simulink model "c960x4096_x14_7_r2013b_frb"  (R2013b)
settings: Solver=ode45  StartTime=0.0  StopTime=40960  RelTol=1e-3
undefined symbols (not defined in the file): sfp
libraries: xbsIndex_r4 x14620, casper_library_misc x61, dspsigops x32, casper_library_multipliers x24, simulink x18, xps_library x18
(part 38 of 79)

== system c960x4096_x14_7_r2013b_frb/vacc/vacc/xx/bit_sel2 ==
  shift : Inport
  sync : Inport  Port=2
  din64 : Inport  Port=3
  Reinterpret : xbsIndex_r4/Reinterpret  force_arith_type=on  arith_type=Unsigned  force_bin_pt=on  bin_pt=0  block_type=reinterpret
  barrel_switcher : Subsystem  AncestorBlock=casper_library_reorder/barrel_switcher  mask(barrel_switcher){n_inputs=6, async=off}
      mask prompts: n_inputs "Number of Inputs: (2^?)"; async "Asynchronous operation"
      mask help:
      | Shifts input to right by amount specified on sel,
      | wrapping around into higher order bits.
      mask init:
      | barrel_switcher_init(gcb,...
      |     'n_inputs', n_inputs, ...
      |     'async', async);
      mask Help: eval('xlWeb(''http://casper.berkeley.edu/wiki/Barrel_switcher'')')
  bus_create : Subsystem  AncestorBlock=casper_library_flow_control/bus_create  mask(bus_create){inputNum=8}
      mask prompts: inputNum "Number of inputs:"
      mask init:
      | bus_create_init(gcb,...
      |     'inputNum', inputNum);
  bus_expand1 : Subsystem  AncestorBlock=casper_library_flow_control/bus_expand  mask(bus_expand){mode=divisions of equal size, outputNum=64, outputWidth=1, outputBinaryPt=0, outputArithmeticType=0, show_format=off, outputToWorkspace=off, variablePrefix=out, outputToModelAsWell=on}
      mask prompts: outputNum "Number of outputs:"; outputWidth "Output width:"; outputBinaryPt "Output binary point position:"; outputArithmeticType "Output arithmetic type (ufix=0, fix=1, bool=2):"; show_format "Print format string?"; outputToWorkspace "Output to workspace?"; variablePrefix "Variable name prefix:"; outputToModelAsWell "Output to model as well?"
      mask help:
      | Expands a 'bus' made using a bus_create or Xilinx
      | concat block.
      | The input will be divided into the specified number
      | of outputs with the specified arithmetic types.
      | Divisions are made from most significant bit.
      mask init: same as c960x4096_x14_7_r2013b_frb/ssg/bus_expand
      settings: AttributesFormatString=64 outputs
      mask TypeOptions mode: divisions of equal size | divisions of arbitrary size
      mask Callback mode: bus_expand_callback();
      mask Callback outputWidth: bus_expand_callback();
      mask Callback outputToWorkspace: bus_expand_callback();
  sync_out : Outport
  dout16 : Outport  Port=2
  wires:
  bus_expand1/13(out52) -> barrel_switcher/15(In13)
  bus_expand1/42(out23) -> barrel_switcher/44(In42)
  bus_expand1/27(out38) -> barrel_switcher/29(In27)
  bus_expand1/26(out39) -> barrel_switcher/28(In26)
  bus_expand1/33(out32) -> barrel_switcher/35(In33)
  bus_expand1/44(out21) -> barrel_switcher/46(In44)
  bus_expand1/12(out53) -> barrel_switcher/14(In12)
  bus_expand1/35(out30) -> barrel_switcher/37(In35)
  bus_expand1/23(out42) -> barrel_switcher/25(In23)
  bus_expand1/45(out20) -> barrel_switcher/47(In45)
  bus_expand1/50(out15) -> barrel_switcher/52(In50)
  bus_expand1/56(out9) -> barrel_switcher/58(In56)
  sync/1 -> barrel_switcher/2(sync_in)
  bus_expand1/24(out41) -> barrel_switcher/26(In24)
  bus_expand1/58(out7) -> barrel_switcher/60(In58)
  bus_expand1/53(out12) -> barrel_switcher/55(In53)
  bus_expand1/29(out36) -> barrel_switcher/31(In29)
  bus_expand1/43(out22) -> barrel_switcher/45(In43)
  bus_expand1/3(out62) -> barrel_switcher/5(In3)
  bus_expand1/61(out4) -> barrel_switcher/63(In61)
  bus_expand1/1(msb_out64) -> barrel_switcher/3(In1)
  bus_expand1/28(out37) -> barrel_switcher/30(In28)
  Reinterpret/1 -> bus_expand1/1(bus_in)
  bus_expand1/8(out57) -> barrel_switcher/10(In8)
  bus_expand1/20(out45) -> barrel_switcher/22(In20)
  bus_expand1/59(out6) -> barrel_switcher/61(In59)
  bus_expand1/30(out35) -> barrel_switcher/32(In30)
  bus_expand1/19(out46) -> barrel_switcher/21(In19)
  bus_expand1/9(out56) -> barrel_switcher/11(In9)
  bus_expand1/11(out54) -> barrel_switcher/13(In11)
  bus_expand1/18(out47) -> barrel_switcher/20(In18)
  bus_expand1/25(out40) -> barrel_switcher/27(In25)
  bus_expand1/32(out33) -> barrel_switcher/34(In32)
  bus_expand1/62(out3) -> barrel_switcher/64(In62)
  bus_expand1/37(out28) -> barrel_switcher/39(In37)
  bus_expand1/36(out29) -> barrel_switcher/38(In36)
  bus_expand1/41(out24) -> barrel_switcher/43(In41)
  bus_expand1/22(out43) -> barrel_switcher/24(In22)
  bus_expand1/48(out17) -> barrel_switcher/50(In48)
  bus_expand1/7(out58) -> barrel_switcher/9(In7)
  bus_expand1/63(out2) -> barrel_switcher/65(In63)
  bus_expand1/15(out50) -> barrel_switcher/17(In15)
  bus_expand1/49(out16) -> barrel_switcher/51(In49)
  shift/1 -> barrel_switcher/1(sel)
  bus_expand1/21(out44) -> barrel_switcher/23(In21)
  bus_expand1/46(out19) -> barrel_switcher/48(In46)
  bus_expand1/52(out13) -> barrel_switcher/54(In52)
  bus_expand1/54(out11) -> barrel_switcher/56(In54)
  bus_expand1/4(out61) -> barrel_switcher/6(In4)
  bus_expand1/31(out34) -> barrel_switcher/33(In31)
  bus_expand1/40(out25) -> barrel_switcher/42(In40)
  bus_expand1/39(out26) -> barrel_switcher/41(In39)
  bus_expand1/51(out14) -> barrel_switcher/53(In51)
  bus_expand1/64(lsb_out1) -> barrel_switcher/66(In64)
  bus_expand1/38(out27) -> barrel_switcher/40(In38)
  din64/1 -> Reinterpret/1
  bus_expand1/5(out60) -> barrel_switcher/7(In5)
  bus_expand1/17(out48) -> barrel_switcher/19(In17)
  bus_expand1/16(out49) -> barrel_switcher/18(In16)
  bus_expand1/10(out55) -> barrel_switcher/12(In10)
  bus_expand1/14(out51) -> barrel_switcher/16(In14)
  bus_expand1/2(out63) -> barrel_switcher/4(In2)
  bus_expand1/60(out5) -> barrel_switcher/62(In60)
  bus_expand1/55(out10) -> barrel_switcher/57(In55)
  bus_expand1/6(out59) -> barrel_switcher/8(In6)
  bus_expand1/47(out18) -> barrel_switcher/49(In47)
  bus_expand1/57(out8) -> barrel_switcher/59(In57)
  bus_expand1/34(out31) -> barrel_switcher/36(In34)
  barrel_switcher/1(sync_out) -> sync_out/1
  bus_create/1(bus_out) -> dout16/1
  barrel_switcher/58(Out57) -> bus_create/1(in1)
  barrel_switcher/59(Out58) -> bus_create/2(in2)
  barrel_switcher/60(Out59) -> bus_create/3(in3)
  barrel_switcher/61(Out60) -> bus_create/4(in4)
  barrel_switcher/62(Out61) -> bus_create/5(in5)
  barrel_switcher/63(Out62) -> bus_create/6(in6)
  barrel_switcher/64(Out63) -> bus_create/7(in7)
  barrel_switcher/65(Out64) -> bus_create/8(in8)

== system c960x4096_x14_7_r2013b_frb/vacc/vacc/xx/bit_sel3 ==
  shift : Inport
  sync : Inport  Port=2
  din64 : Inport  Port=3
  Reinterpret : xbsIndex_r4/Reinterpret  force_arith_type=on  arith_type=Unsigned  force_bin_pt=on  bin_pt=0  block_type=reinterpret
  barrel_switcher : Subsystem  AncestorBlock=casper_library_reorder/barrel_switcher  mask(barrel_switcher){n_inputs=6, async=off}
      mask prompts: n_inputs "Number of Inputs: (2^?)"; async "Asynchronous operation"
      mask help:
      | Shifts input to right by amount specified on sel,
      | wrapping around into higher order bits.
      mask init:
      | barrel_switcher_init(gcb,...
      |     'n_inputs', n_inputs, ...
      |     'async', async);
      mask Help: eval('xlWeb(''http://casper.berkeley.edu/wiki/Barrel_switcher'')')
  bus_create : Subsystem  AncestorBlock=casper_library_flow_control/bus_create  mask(bus_create){inputNum=8}
      mask prompts: inputNum "Number of inputs:"
      mask init:
      | bus_create_init(gcb,...
      |     'inputNum', inputNum);
  bus_expand1 : Subsystem  AncestorBlock=casper_library_flow_control/bus_expand  mask(bus_expand){mode=divisions of equal size, outputNum=64, outputWidth=1, outputBinaryPt=0, outputArithmeticType=0, show_format=off, outputToWorkspace=off, variablePrefix=out, outputToModelAsWell=on}
      mask prompts: outputNum "Number of outputs:"; outputWidth "Output width:"; outputBinaryPt "Output binary point position:"; outputArithmeticType "Output arithmetic type (ufix=0, fix=1, bool=2):"; show_format "Print format string?"; outputToWorkspace "Output to workspace?"; variablePrefix "Variable name prefix:"; outputToModelAsWell "Output to model as well?"
      mask help:
      | Expands a 'bus' made using a bus_create or Xilinx
      | concat block.
      | The input will be divided into the specified number
      | of outputs with the specified arithmetic types.
      | Divisions are made from most significant bit.
      mask init: same as c960x4096_x14_7_r2013b_frb/ssg/bus_expand
      settings: AttributesFormatString=64 outputs
      mask TypeOptions mode: divisions of equal size | divisions of arbitrary size
      mask Callback mode: bus_expand_callback();
      mask Callback outputWidth: bus_expand_callback();
      mask Callback outputToWorkspace: bus_expand_callback();
  sync_out : Outport
  dout16 : Outport  Port=2
  wires:
  bus_expand1/13(out52) -> barrel_switcher/15(In13)
  bus_expand1/42(out23) -> barrel_switcher/44(In42)
  bus_expand1/27(out38) -> barrel_switcher/29(In27)
  bus_expand1/26(out39) -> barrel_switcher/28(In26)
  bus_expand1/33(out32) -> barrel_switcher/35(In33)
  bus_expand1/44(out21) -> barrel_switcher/46(In44)
  bus_expand1/12(out53) -> barrel_switcher/14(In12)
  bus_expand1/35(out30) -> barrel_switcher/37(In35)
  bus_expand1/23(out42) -> barrel_switcher/25(In23)
  bus_expand1/45(out20) -> barrel_switcher/47(In45)
  bus_expand1/50(out15) -> barrel_switcher/52(In50)
  bus_expand1/56(out9) -> barrel_switcher/58(In56)
  sync/1 -> barrel_switcher/2(sync_in)
  bus_expand1/24(out41) -> barrel_switcher/26(In24)
  bus_expand1/58(out7) -> barrel_switcher/60(In58)
  bus_expand1/53(out12) -> barrel_switcher/55(In53)
  bus_expand1/29(out36) -> barrel_switcher/31(In29)
  bus_expand1/43(out22) -> barrel_switcher/45(In43)
  bus_expand1/3(out62) -> barrel_switcher/5(In3)
  bus_expand1/61(out4) -> barrel_switcher/63(In61)
  bus_expand1/1(msb_out64) -> barrel_switcher/3(In1)
  bus_expand1/28(out37) -> barrel_switcher/30(In28)
  Reinterpret/1 -> bus_expand1/1(bus_in)
  bus_expand1/8(out57) -> barrel_switcher/10(In8)
  bus_expand1/20(out45) -> barrel_switcher/22(In20)
  bus_expand1/59(out6) -> barrel_switcher/61(In59)
  bus_expand1/30(out35) -> barrel_switcher/32(In30)
  bus_expand1/19(out46) -> barrel_switcher/21(In19)
  bus_expand1/9(out56) -> barrel_switcher/11(In9)
  bus_expand1/11(out54) -> barrel_switcher/13(In11)
  bus_expand1/18(out47) -> barrel_switcher/20(In18)
  bus_expand1/25(out40) -> barrel_switcher/27(In25)
  bus_expand1/32(out33) -> barrel_switcher/34(In32)
  bus_expand1/62(out3) -> barrel_switcher/64(In62)
  bus_expand1/37(out28) -> barrel_switcher/39(In37)
  bus_expand1/36(out29) -> barrel_switcher/38(In36)
  bus_expand1/41(out24) -> barrel_switcher/43(In41)
  bus_expand1/22(out43) -> barrel_switcher/24(In22)
  bus_expand1/48(out17) -> barrel_switcher/50(In48)
  bus_expand1/7(out58) -> barrel_switcher/9(In7)
  bus_expand1/63(out2) -> barrel_switcher/65(In63)
  bus_expand1/15(out50) -> barrel_switcher/17(In15)
  bus_expand1/49(out16) -> barrel_switcher/51(In49)
  shift/1 -> barrel_switcher/1(sel)
  bus_expand1/21(out44) -> barrel_switcher/23(In21)
  bus_expand1/46(out19) -> barrel_switcher/48(In46)
  bus_expand1/52(out13) -> barrel_switcher/54(In52)
  bus_expand1/54(out11) -> barrel_switcher/56(In54)
  bus_expand1/4(out61) -> barrel_switcher/6(In4)
  bus_expand1/31(out34) -> barrel_switcher/33(In31)
  bus_expand1/40(out25) -> barrel_switcher/42(In40)
  bus_expand1/39(out26) -> barrel_switcher/41(In39)
  bus_expand1/51(out14) -> barrel_switcher/53(In51)
  bus_expand1/64(lsb_out1) -> barrel_switcher/66(In64)
  bus_expand1/38(out27) -> barrel_switcher/40(In38)
  din64/1 -> Reinterpret/1
  bus_expand1/5(out60) -> barrel_switcher/7(In5)
  bus_expand1/17(out48) -> barrel_switcher/19(In17)
  bus_expand1/16(out49) -> barrel_switcher/18(In16)
  bus_expand1/10(out55) -> barrel_switcher/12(In10)
  bus_expand1/14(out51) -> barrel_switcher/16(In14)
  bus_expand1/2(out63) -> barrel_switcher/4(In2)
  bus_expand1/60(out5) -> barrel_switcher/62(In60)
  bus_expand1/55(out10) -> barrel_switcher/57(In55)
  bus_expand1/6(out59) -> barrel_switcher/8(In6)
  bus_expand1/47(out18) -> barrel_switcher/49(In47)
  bus_expand1/57(out8) -> barrel_switcher/59(In57)
  bus_expand1/34(out31) -> barrel_switcher/36(In34)
  barrel_switcher/1(sync_out) -> sync_out/1
  bus_create/1(bus_out) -> dout16/1
  barrel_switcher/58(Out57) -> bus_create/1(in1)
  barrel_switcher/59(Out58) -> bus_create/2(in2)
  barrel_switcher/60(Out59) -> bus_create/3(in3)
  barrel_switcher/61(Out60) -> bus_create/4(in4)
  barrel_switcher/62(Out61) -> bus_create/5(in5)
  barrel_switcher/63(Out62) -> bus_create/6(in6)
  barrel_switcher/64(Out63) -> bus_create/7(in7)
  barrel_switcher/65(Out64) -> bus_create/8(in8)

== system c960x4096_x14_7_r2013b_frb/vacc/vacc/xx/bit_sel4 ==
  shift : Inport
  sync : Inport  Port=2
  din64 : Inport  Port=3
  Reinterpret : xbsIndex_r4/Reinterpret  force_arith_type=on  arith_type=Unsigned  force_bin_pt=on  bin_pt=0  block_type=reinterpret
  barrel_switcher : Subsystem  AncestorBlock=casper_library_reorder/barrel_switcher  mask(barrel_switcher){n_inputs=6, async=off}
      mask prompts: n_inputs "Number of Inputs: (2^?)"; async "Asynchronous operation"
      mask help:
      | Shifts input to right by amount specified on sel,
      | wrapping around into higher order bits.
      mask init:
      | barrel_switcher_init(gcb,...
      |     'n_inputs', n_inputs, ...
      |     'async', async);
      mask Help: eval('xlWeb(''http://casper.berkeley.edu/wiki/Barrel_switcher'')')
  bus_create : Subsystem  AncestorBlock=casper_library_flow_control/bus_create  mask(bus_create){inputNum=8}
      mask prompts: inputNum "Number of inputs:"
      mask init:
      | bus_create_init(gcb,...
      |     'inputNum', inputNum);
  bus_expand1 : Subsystem  AncestorBlock=casper_library_flow_control/bus_expand  mask(bus_expand){mode=divisions of equal size, outputNum=64, outputWidth=1, outputBinaryPt=0, outputArithmeticType=0, show_format=off, outputToWorkspace=off, variablePrefix=out, outputToModelAsWell=on}
      mask prompts: outputNum "Number of outputs:"; outputWidth "Output width:"; outputBinaryPt "Output binary point position:"; outputArithmeticType "Output arithmetic type (ufix=0, fix=1, bool=2):"; show_format "Print format string?"; outputToWorkspace "Output to workspace?"; variablePrefix "Variable name prefix:"; outputToModelAsWell "Output to model as well?"
      mask help:
      | Expands a 'bus' made using a bus_create or Xilinx
      | concat block.
      | The input will be divided into the specified number
      | of outputs with the specified arithmetic types.
      | Divisions are made from most significant bit.
      mask init: same as c960x4096_x14_7_r2013b_frb/ssg/bus_expand
      settings: AttributesFormatString=64 outputs
      mask TypeOptions mode: divisions of equal size | divisions of arbitrary size
      mask Callback mode: bus_expand_callback();
      mask Callback outputWidth: bus_expand_callback();
      mask Callback outputToWorkspace: bus_expand_callback();
  sync_out : Outport
  dout16 : Outport  Port=2
  wires:
  bus_expand1/13(out52) -> barrel_switcher/15(In13)
  bus_expand1/42(out23) -> barrel_switcher/44(In42)
  bus_expand1/27(out38) -> barrel_switcher/29(In27)
  bus_expand1/26(out39) -> barrel_switcher/28(In26)
  bus_expand1/33(out32) -> barrel_switcher/35(In33)
  bus_expand1/44(out21) -> barrel_switcher/46(In44)
  bus_expand1/12(out53) -> barrel_switcher/14(In12)
  bus_expand1/35(out30) -> barrel_switcher/37(In35)
  bus_expand1/23(out42) -> barrel_switcher/25(In23)
  bus_expand1/45(out20) -> barrel_switcher/47(In45)
  bus_expand1/50(out15) -> barrel_switcher/52(In50)
  bus_expand1/56(out9) -> barrel_switcher/58(In56)
  sync/1 -> barrel_switcher/2(sync_in)
  bus_expand1/24(out41) -> barrel_switcher/26(In24)
  bus_expand1/58(out7) -> barrel_switcher/60(In58)
  bus_expand1/53(out12) -> barrel_switcher/55(In53)
  bus_expand1/29(out36) -> barrel_switcher/31(In29)
  bus_expand1/43(out22) -> barrel_switcher/45(In43)
  bus_expand1/3(out62) -> barrel_switcher/5(In3)
  bus_expand1/61(out4) -> barrel_switcher/63(In61)
  bus_expand1/1(msb_out64) -> barrel_switcher/3(In1)
  bus_expand1/28(out37) -> barrel_switcher/30(In28)
  Reinterpret/1 -> bus_expand1/1(bus_in)
  bus_expand1/8(out57) -> barrel_switcher/10(In8)
  bus_expand1/20(out45) -> barrel_switcher/22(In20)
  bus_expand1/59(out6) -> barrel_switcher/61(In59)
  bus_expand1/30(out35) -> barrel_switcher/32(In30)
  bus_expand1/19(out46) -> barrel_switcher/21(In19)
  bus_expand1/9(out56) -> barrel_switcher/11(In9)
  bus_expand1/11(out54) -> barrel_switcher/13(In11)
  bus_expand1/18(out47) -> barrel_switcher/20(In18)
  bus_expand1/25(out40) -> barrel_switcher/27(In25)
  bus_expand1/32(out33) -> barrel_switcher/34(In32)
  bus_expand1/62(out3) -> barrel_switcher/64(In62)
  bus_expand1/37(out28) -> barrel_switcher/39(In37)
  bus_expand1/36(out29) -> barrel_switcher/38(In36)
  bus_expand1/41(out24) -> barrel_switcher/43(In41)
  bus_expand1/22(out43) -> barrel_switcher/24(In22)
  bus_expand1/48(out17) -> barrel_switcher/50(In48)
  bus_expand1/7(out58) -> barrel_switcher/9(In7)
  bus_expand1/63(out2) -> barrel_switcher/65(In63)
  bus_expand1/15(out50) -> barrel_switcher/17(In15)
  bus_expand1/49(out16) -> barrel_switcher/51(In49)
  shift/1 -> barrel_switcher/1(sel)
  bus_expand1/21(out44) -> barrel_switcher/23(In21)
  bus_expand1/46(out19) -> barrel_switcher/48(In46)
  bus_expand1/52(out13) -> barrel_switcher/54(In52)
  bus_expand1/54(out11) -> barrel_switcher/56(In54)
  bus_expand1/4(out61) -> barrel_switcher/6(In4)
  bus_expand1/31(out34) -> barrel_switcher/33(In31)
  bus_expand1/40(out25) -> barrel_switcher/42(In40)
  bus_expand1/39(out26) -> barrel_switcher/41(In39)
  bus_expand1/51(out14) -> barrel_switcher/53(In51)
  bus_expand1/64(lsb_out1) -> barrel_switcher/66(In64)
  bus_expand1/38(out27) -> barrel_switcher/40(In38)
  din64/1 -> Reinterpret/1
  bus_expand1/5(out60) -> barrel_switcher/7(In5)
  bus_expand1/17(out48) -> barrel_switcher/19(In17)
  bus_expand1/16(out49) -> barrel_switcher/18(In16)
  bus_expand1/10(out55) -> barrel_switcher/12(In10)
  bus_expand1/14(out51) -> barrel_switcher/16(In14)
  bus_expand1/2(out63) -> barrel_switcher/4(In2)
  bus_expand1/60(out5) -> barrel_switcher/62(In60)
  bus_expand1/55(out10) -> barrel_switcher/57(In55)
  bus_expand1/6(out59) -> barrel_switcher/8(In6)
  bus_expand1/47(out18) -> barrel_switcher/49(In47)
  bus_expand1/57(out8) -> barrel_switcher/59(In57)
  bus_expand1/34(out31) -> barrel_switcher/36(In34)
  barrel_switcher/1(sync_out) -> sync_out/1
  bus_create/1(bus_out) -> dout16/1
  barrel_switcher/58(Out57) -> bus_create/1(in1)
  barrel_switcher/59(Out58) -> bus_create/2(in2)
  barrel_switcher/60(Out59) -> bus_create/3(in3)
  barrel_switcher/61(Out60) -> bus_create/4(in4)
  barrel_switcher/62(Out61) -> bus_create/5(in5)
  barrel_switcher/63(Out62) -> bus_create/6(in6)
  barrel_switcher/64(Out63) -> bus_create/7(in7)
  barrel_switcher/65(Out64) -> bus_create/8(in8)

== system c960x4096_x14_7_r2013b_frb/vacc/vacc/xx/bit_sel5 ==
  shift : Inport
  sync : Inport  Port=2
  din64 : Inport  Port=3
  Reinterpret : xbsIndex_r4/Reinterpret  force_arith_type=on  arith_type=Unsigned  force_bin_pt=on  bin_pt=0  block_type=reinterpret
  barrel_switcher : Subsystem  AncestorBlock=casper_library_reorder/barrel_switcher  mask(barrel_switcher){n_inputs=6, async=off}
      mask prompts: n_inputs "Number of Inputs: (2^?)"; async "Asynchronous operation"
      mask help:
      | Shifts input to right by amount specified on sel,
      | wrapping around into higher order bits.
      mask init:
      | barrel_switcher_init(gcb,...
      |     'n_inputs', n_inputs, ...
      |     'async', async);
      mask Help: eval('xlWeb(''http://casper.berkeley.edu/wiki/Barrel_switcher'')')
  bus_create : Subsystem  AncestorBlock=casper_library_flow_control/bus_create  mask(bus_create){inputNum=8}
      mask prompts: inputNum "Number of inputs:"
      mask init:
      | bus_create_init(gcb,...
      |     'inputNum', inputNum);
  bus_expand1 : Subsystem  AncestorBlock=casper_library_flow_control/bus_expand  mask(bus_expand){mode=divisions of equal size, outputNum=64, outputWidth=1, outputBinaryPt=0, outputArithmeticType=0, show_format=off, outputToWorkspace=off, variablePrefix=out, outputToModelAsWell=on}
      mask prompts: outputNum "Number of outputs:"; outputWidth "Output width:"; outputBinaryPt "Output binary point position:"; outputArithmeticType "Output arithmetic type (ufix=0, fix=1, bool=2):"; show_format "Print format string?"; outputToWorkspace "Output to workspace?"; variablePrefix "Variable name prefix:"; outputToModelAsWell "Output to model as well?"
      mask help:
      | Expands a 'bus' made using a bus_create or Xilinx
      | concat block.
      | The input will be divided into the specified number
      | of outputs with the specified arithmetic types.
      | Divisions are made from most significant bit.
      mask init: same as c960x4096_x14_7_r2013b_frb/ssg/bus_expand
      settings: AttributesFormatString=64 outputs
      mask TypeOptions mode: divisions of equal size | divisions of arbitrary size
      mask Callback mode: bus_expand_callback();
      mask Callback outputWidth: bus_expand_callback();
      mask Callback outputToWorkspace: bus_expand_callback();
  sync_out : Outport
  dout16 : Outport  Port=2
  wires:
  bus_expand1/13(out52) -> barrel_switcher/15(In13)
  bus_expand1/42(out23) -> barrel_switcher/44(In42)
  bus_expand1/27(out38) -> barrel_switcher/29(In27)
  bus_expand1/26(out39) -> barrel_switcher/28(In26)
  bus_expand1/33(out32) -> barrel_switcher/35(In33)
  bus_expand1/44(out21) -> barrel_switcher/46(In44)
  bus_expand1/12(out53) -> barrel_switcher/14(In12)
  bus_expand1/35(out30) -> barrel_switcher/37(In35)
  bus_expand1/23(out42) -> barrel_switcher/25(In23)
  bus_expand1/45(out20) -> barrel_switcher/47(In45)
  bus_expand1/50(out15) -> barrel_switcher/52(In50)
  bus_expand1/56(out9) -> barrel_switcher/58(In56)
  sync/1 -> barrel_switcher/2(sync_in)
  bus_expand1/24(out41) -> barrel_switcher/26(In24)
  bus_expand1/58(out7) -> barrel_switcher/60(In58)
  bus_expand1/53(out12) -> barrel_switcher/55(In53)
  bus_expand1/29(out36) -> barrel_switcher/31(In29)
  bus_expand1/43(out22) -> barrel_switcher/45(In43)
  bus_expand1/3(out62) -> barrel_switcher/5(In3)
  bus_expand1/61(out4) -> barrel_switcher/63(In61)
  bus_expand1/1(msb_out64) -> barrel_switcher/3(In1)
  bus_expand1/28(out37) -> barrel_switcher/30(In28)
  Reinterpret/1 -> bus_expand1/1(bus_in)
  bus_expand1/8(out57) -> barrel_switcher/10(In8)
  bus_expand1/20(out45) -> barrel_switcher/22(In20)
  bus_expand1/59(out6) -> barrel_switcher/61(In59)
  bus_expand1/30(out35) -> barrel_switcher/32(In30)
  bus_expand1/19(out46) -> barrel_switcher/21(In19)
  bus_expand1/9(out56) -> barrel_switcher/11(In9)
  bus_expand1/11(out54) -> barrel_switcher/13(In11)
  bus_expand1/18(out47) -> barrel_switcher/20(In18)
  bus_expand1/25(out40) -> barrel_switcher/27(In25)
  bus_expand1/32(out33) -> barrel_switcher/34(In32)
  bus_expand1/62(out3) -> barrel_switcher/64(In62)
  bus_expand1/37(out28) -> barrel_switcher/39(In37)
  bus_expand1/36(out29) -> barrel_switcher/38(In36)
  bus_expand1/41(out24) -> barrel_switcher/43(In41)
  bus_expand1/22(out43) -> barrel_switcher/24(In22)
  bus_expand1/48(out17) -> barrel_switcher/50(In48)
  bus_expand1/7(out58) -> barrel_switcher/9(In7)
  bus_expand1/63(out2) -> barrel_switcher/65(In63)
  bus_expand1/15(out50) -> barrel_switcher/17(In15)
  bus_expand1/49(out16) -> barrel_switcher/51(In49)
  shift/1 -> barrel_switcher/1(sel)
  bus_expand1/21(out44) -> barrel_switcher/23(In21)
  bus_expand1/46(out19) -> barrel_switcher/48(In46)
  bus_expand1/52(out13) -> barrel_switcher/54(In52)
  bus_expand1/54(out11) -> barrel_switcher/56(In54)
  bus_expand1/4(out61) -> barrel_switcher/6(In4)
  bus_expand1/31(out34) -> barrel_switcher/33(In31)
  bus_expand1/40(out25) -> barrel_switcher/42(In40)
  bus_expand1/39(out26) -> barrel_switcher/41(In39)
  bus_expand1/51(out14) -> barrel_switcher/53(In51)
  bus_expand1/64(lsb_out1) -> barrel_switcher/66(In64)
  bus_expand1/38(out27) -> barrel_switcher/40(In38)
  din64/1 -> Reinterpret/1
  bus_expand1/5(out60) -> barrel_switcher/7(In5)
  bus_expand1/17(out48) -> barrel_switcher/19(In17)
  bus_expand1/16(out49) -> barrel_switcher/18(In16)
  bus_expand1/10(out55) -> barrel_switcher/12(In10)
  bus_expand1/14(out51) -> barrel_switcher/16(In14)
  bus_expand1/2(out63) -> barrel_switcher/4(In2)
  bus_expand1/60(out5) -> barrel_switcher/62(In60)
  bus_expand1/55(out10) -> barrel_switcher/57(In55)
  bus_expand1/6(out59) -> barrel_switcher/8(In6)
  bus_expand1/47(out18) -> barrel_switcher/49(In47)
  bus_expand1/57(out8) -> barrel_switcher/59(In57)
  bus_expand1/34(out31) -> barrel_switcher/36(In34)
  barrel_switcher/1(sync_out) -> sync_out/1
  bus_create/1(bus_out) -> dout16/1
  barrel_switcher/58(Out57) -> bus_create/1(in1)
  barrel_switcher/59(Out58) -> bus_create/2(in2)
  barrel_switcher/60(Out59) -> bus_create/3(in3)
  barrel_switcher/61(Out60) -> bus_create/4(in4)
  barrel_switcher/62(Out61) -> bus_create/5(in5)
  barrel_switcher/63(Out62) -> bus_create/6(in6)
  barrel_switcher/64(Out63) -> bus_create/7(in7)
  barrel_switcher/65(Out64) -> bus_create/8(in8)

== system c960x4096_x14_7_r2013b_frb/vacc/vacc/xx/bit_sel6 ==
  shift : Inport
  sync : Inport  Port=2
  din64 : Inport  Port=3
  Reinterpret : xbsIndex_r4/Reinterpret  force_arith_type=on  arith_type=Unsigned  force_bin_pt=on  bin_pt=0  block_type=reinterpret
  barrel_switcher : Subsystem  AncestorBlock=casper_library_reorder/barrel_switcher  mask(barrel_switcher){n_inputs=6, async=off}
      mask prompts: n_inputs "Number of Inputs: (2^?)"; async "Asynchronous operation"
      mask help:
      | Shifts input to right by amount specified on sel,
      | wrapping around into higher order bits.
      mask init:
      | barrel_switcher_init(gcb,...
      |     'n_inputs', n_inputs, ...
      |     'async', async);
      mask Help: eval('xlWeb(''http://casper.berkeley.edu/wiki/Barrel_switcher'')')
  bus_create : Subsystem  AncestorBlock=casper_library_flow_control/bus_create  mask(bus_create){inputNum=8}
      mask prompts: inputNum "Number of inputs:"
      mask init:
      | bus_create_init(gcb,...
      |     'inputNum', inputNum);
  bus_expand1 : Subsystem  AncestorBlock=casper_library_flow_control/bus_expand  mask(bus_expand){mode=divisions of equal size, outputNum=64, outputWidth=1, outputBinaryPt=0, outputArithmeticType=0, show_format=off, outputToWorkspace=off, variablePrefix=out, outputToModelAsWell=on}
      mask prompts: outputNum "Number of outputs:"; outputWidth "Output width:"; outputBinaryPt "Output binary point position:"; outputArithmeticType "Output arithmetic type (ufix=0, fix=1, bool=2):"; show_format "Print format string?"; outputToWorkspace "Output to workspace?"; variablePrefix "Variable name prefix:"; outputToModelAsWell "Output to model as well?"
      mask help:
      | Expands a 'bus' made using a bus_create or Xilinx
      | concat block.
      | The input will be divided into the specified number
      | of outputs with the specified arithmetic types.
      | Divisions are made from most significant bit.
      mask init: same as c960x4096_x14_7_r2013b_frb/ssg/bus_expand
      settings: AttributesFormatString=64 outputs
      mask TypeOptions mode: divisions of equal size | divisions of arbitrary size
      mask Callback mode: bus_expand_callback();
      mask Callback outputWidth: bus_expand_callback();
      mask Callback outputToWorkspace: bus_expand_callback();
  sync_out : Outport
  dout16 : Outport  Port=2
  wires:
  bus_expand1/13(out52) -> barrel_switcher/15(In13)
  bus_expand1/42(out23) -> barrel_switcher/44(In42)
  bus_expand1/27(out38) -> barrel_switcher/29(In27)
  bus_expand1/26(out39) -> barrel_switcher/28(In26)
  bus_expand1/33(out32) -> barrel_switcher/35(In33)
  bus_expand1/44(out21) -> barrel_switcher/46(In44)
  bus_expand1/12(out53) -> barrel_switcher/14(In12)
  bus_expand1/35(out30) -> barrel_switcher/37(In35)
  bus_expand1/23(out42) -> barrel_switcher/25(In23)
  bus_expand1/45(out20) -> barrel_switcher/47(In45)
  bus_expand1/50(out15) -> barrel_switcher/52(In50)
  bus_expand1/56(out9) -> barrel_switcher/58(In56)
  sync/1 -> barrel_switcher/2(sync_in)
  bus_expand1/24(out41) -> barrel_switcher/26(In24)
  bus_expand1/58(out7) -> barrel_switcher/60(In58)
  bus_expand1/53(out12) -> barrel_switcher/55(In53)
  bus_expand1/29(out36) -> barrel_switcher/31(In29)
  bus_expand1/43(out22) -> barrel_switcher/45(In43)
  bus_expand1/3(out62) -> barrel_switcher/5(In3)
  bus_expand1/61(out4) -> barrel_switcher/63(In61)
  bus_expand1/1(msb_out64) -> barrel_switcher/3(In1)
  bus_expand1/28(out37) -> barrel_switcher/30(In28)
  Reinterpret/1 -> bus_expand1/1(bus_in)
  bus_expand1/8(out57) -> barrel_switcher/10(In8)
  bus_expand1/20(out45) -> barrel_switcher/22(In20)
  bus_expand1/59(out6) -> barrel_switcher/61(In59)
  bus_expand1/30(out35) -> barrel_switcher/32(In30)
  bus_expand1/19(out46) -> barrel_switcher/21(In19)
  bus_expand1/9(out56) -> barrel_switcher/11(In9)
  bus_expand1/11(out54) -> barrel_switcher/13(In11)
  bus_expand1/18(out47) -> barrel_switcher/20(In18)
  bus_expand1/25(out40) -> barrel_switcher/27(In25)
  bus_expand1/32(out33) -> barrel_switcher/34(In32)
  bus_expand1/62(out3) -> barrel_switcher/64(In62)
  bus_expand1/37(out28) -> barrel_switcher/39(In37)
  bus_expand1/36(out29) -> barrel_switcher/38(In36)
  bus_expand1/41(out24) -> barrel_switcher/43(In41)
  bus_expand1/22(out43) -> barrel_switcher/24(In22)
  bus_expand1/48(out17) -> barrel_switcher/50(In48)
  bus_expand1/7(out58) -> barrel_switcher/9(In7)
  bus_expand1/63(out2) -> barrel_switcher/65(In63)
  bus_expand1/15(out50) -> barrel_switcher/17(In15)
  bus_expand1/49(out16) -> barrel_switcher/51(In49)
  shift/1 -> barrel_switcher/1(sel)
  bus_expand1/21(out44) -> barrel_switcher/23(In21)
  bus_expand1/46(out19) -> barrel_switcher/48(In46)
  bus_expand1/52(out13) -> barrel_switcher/54(In52)
  bus_expand1/54(out11) -> barrel_switcher/56(In54)
  bus_expand1/4(out61) -> barrel_switcher/6(In4)
  bus_expand1/31(out34) -> barrel_switcher/33(In31)
  bus_expand1/40(out25) -> barrel_switcher/42(In40)
  bus_expand1/39(out26) -> barrel_switcher/41(In39)
  bus_expand1/51(out14) -> barrel_switcher/53(In51)
  bus_expand1/64(lsb_out1) -> barrel_switcher/66(In64)
  bus_expand1/38(out27) -> barrel_switcher/40(In38)
  din64/1 -> Reinterpret/1
  bus_expand1/5(out60) -> barrel_switcher/7(In5)
  bus_expand1/17(out48) -> barrel_switcher/19(In17)
  bus_expand1/16(out49) -> barrel_switcher/18(In16)
  bus_expand1/10(out55) -> barrel_switcher/12(In10)
  bus_expand1/14(out51) -> barrel_switcher/16(In14)
  bus_expand1/2(out63) -> barrel_switcher/4(In2)
  bus_expand1/60(out5) -> barrel_switcher/62(In60)
  bus_expand1/55(out10) -> barrel_switcher/57(In55)
  bus_expand1/6(out59) -> barrel_switcher/8(In6)
  bus_expand1/47(out18) -> barrel_switcher/49(In47)
  bus_expand1/57(out8) -> barrel_switcher/59(In57)
  bus_expand1/34(out31) -> barrel_switcher/36(In34)
  barrel_switcher/1(sync_out) -> sync_out/1
  bus_create/1(bus_out) -> dout16/1
  barrel_switcher/58(Out57) -> bus_create/1(in1)
  barrel_switcher/59(Out58) -> bus_create/2(in2)
  barrel_switcher/60(Out59) -> bus_create/3(in3)
  barrel_switcher/61(Out60) -> bus_create/4(in4)
  barrel_switcher/62(Out61) -> bus_create/5(in5)
  barrel_switcher/63(Out62) -> bus_create/6(in6)
  barrel_switcher/64(Out63) -> bus_create/7(in7)
  barrel_switcher/65(Out64) -> bus_create/8(in8)

== system c960x4096_x14_7_r2013b_frb/vacc/vacc/xx/bit_sel7 ==
  shift : Inport
  sync : Inport  Port=2
  din64 : Inport  Port=3
  Reinterpret : xbsIndex_r4/Reinterpret  force_arith_type=on  arith_type=Unsigned  force_bin_pt=on  bin_pt=0  block_type=reinterpret
  barrel_switcher : Subsystem  AncestorBlock=casper_library_reorder/barrel_switcher  mask(barrel_switcher){n_inputs=6, async=off}
      mask prompts: n_inputs "Number of Inputs: (2^?)"; async "Asynchronous operation"
      mask help:
      | Shifts input to right by amount specified on sel,
      | wrapping around into higher order bits.
      mask init:
      | barrel_switcher_init(gcb,...
      |     'n_inputs', n_inputs, ...
      |     'async', async);
      mask Help: eval('xlWeb(''http://casper.berkeley.edu/wiki/Barrel_switcher'')')
  bus_create : Subsystem  AncestorBlock=casper_library_flow_control/bus_create  mask(bus_create){inputNum=8}
      mask prompts: inputNum "Number of inputs:"
      mask init:
      | bus_create_init(gcb,...
      |     'inputNum', inputNum);
  bus_expand1 : Subsystem  AncestorBlock=casper_library_flow_control/bus_expand  mask(bus_expand){mode=divisions of equal size, outputNum=64, outputWidth=1, outputBinaryPt=0, outputArithmeticType=0, show_format=off, outputToWorkspace=off, variablePrefix=out, outputToModelAsWell=on}
      mask prompts: outputNum "Number of outputs:"; outputWidth "Output width:"; outputBinaryPt "Output binary point position:"; outputArithmeticType "Output arithmetic type (ufix=0, fix=1, bool=2):"; show_format "Print format string?"; outputToWorkspace "Output to workspace?"; variablePrefix "Variable name prefix:"; outputToModelAsWell "Output to model as well?"
      mask help:
      | Expands a 'bus' made using a bus_create or Xilinx
      | concat block.
      | The input will be divided into the specified number
      | of outputs with the specified arithmetic types.
      | Divisions are made from most significant bit.
      mask init: same as c960x4096_x14_7_r2013b_frb/ssg/bus_expand
      settings: AttributesFormatString=64 outputs
      mask TypeOptions mode: divisions of equal size | divisions of arbitrary size
      mask Callback mode: bus_expand_callback();
      mask Callback outputWidth: bus_expand_callback();
      mask Callback outputToWorkspace: bus_expand_callback();
  sync_out : Outport
  dout16 : Outport  Port=2
  wires:
  bus_expand1/13(out52) -> barrel_switcher/15(In13)
  bus_expand1/42(out23) -> barrel_switcher/44(In42)
  bus_expand1/27(out38) -> barrel_switcher/29(In27)
  bus_expand1/26(out39) -> barrel_switcher/28(In26)
  bus_expand1/33(out32) -> barrel_switcher/35(In33)
  bus_expand1/44(out21) -> barrel_switcher/46(In44)
  bus_expand1/12(out53) -> barrel_switcher/14(In12)
  bus_expand1/35(out30) -> barrel_switcher/37(In35)
  bus_expand1/23(out42) -> barrel_switcher/25(In23)
  bus_expand1/45(out20) -> barrel_switcher/47(In45)
  bus_expand1/50(out15) -> barrel_switcher/52(In50)
  bus_expand1/56(out9) -> barrel_switcher/58(In56)
  sync/1 -> barrel_switcher/2(sync_in)
  bus_expand1/24(out41) -> barrel_switcher/26(In24)
  bus_expand1/58(out7) -> barrel_switcher/60(In58)
  bus_expand1/53(out12) -> barrel_switcher/55(In53)
  bus_expand1/29(out36) -> barrel_switcher/31(In29)
  bus_expand1/43(out22) -> barrel_switcher/45(In43)
  bus_expand1/3(out62) -> barrel_switcher/5(In3)
  bus_expand1/61(out4) -> barrel_switcher/63(In61)
  bus_expand1/1(msb_out64) -> barrel_switcher/3(In1)
  bus_expand1/28(out37) -> barrel_switcher/30(In28)
  Reinterpret/1 -> bus_expand1/1(bus_in)
  bus_expand1/8(out57) -> barrel_switcher/10(In8)
  bus_expand1/20(out45) -> barrel_switcher/22(In20)
  bus_expand1/59(out6) -> barrel_switcher/61(In59)
  bus_expand1/30(out35) -> barrel_switcher/32(In30)
  bus_expand1/19(out46) -> barrel_switcher/21(In19)
  bus_expand1/9(out56) -> barrel_switcher/11(In9)
  bus_expand1/11(out54) -> barrel_switcher/13(In11)
  bus_expand1/18(out47) -> barrel_switcher/20(In18)
  bus_expand1/25(out40) -> barrel_switcher/27(In25)
  bus_expand1/32(out33) -> barrel_switcher/34(In32)
  bus_expand1/62(out3) -> barrel_switcher/64(In62)
  bus_expand1/37(out28) -> barrel_switcher/39(In37)
  bus_expand1/36(out29) -> barrel_switcher/38(In36)
  bus_expand1/41(out24) -> barrel_switcher/43(In41)
  bus_expand1/22(out43) -> barrel_switcher/24(In22)
  bus_expand1/48(out17) -> barrel_switcher/50(In48)
  bus_expand1/7(out58) -> barrel_switcher/9(In7)
  bus_expand1/63(out2) -> barrel_switcher/65(In63)
  bus_expand1/15(out50) -> barrel_switcher/17(In15)
  bus_expand1/49(out16) -> barrel_switcher/51(In49)
  shift/1 -> barrel_switcher/1(sel)
  bus_expand1/21(out44) -> barrel_switcher/23(In21)
  bus_expand1/46(out19) -> barrel_switcher/48(In46)
  bus_expand1/52(out13) -> barrel_switcher/54(In52)
  bus_expand1/54(out11) -> barrel_switcher/56(In54)
  bus_expand1/4(out61) -> barrel_switcher/6(In4)
  bus_expand1/31(out34) -> barrel_switcher/33(In31)
  bus_expand1/40(out25) -> barrel_switcher/42(In40)
  bus_expand1/39(out26) -> barrel_switcher/41(In39)
  bus_expand1/51(out14) -> barrel_switcher/53(In51)
  bus_expand1/64(lsb_out1) -> barrel_switcher/66(In64)
  bus_expand1/38(out27) -> barrel_switcher/40(In38)
  din64/1 -> Reinterpret/1
  bus_expand1/5(out60) -> barrel_switcher/7(In5)
  bus_expand1/17(out48) -> barrel_switcher/19(In17)
  bus_expand1/16(out49) -> barrel_switcher/18(In16)
  bus_expand1/10(out55) -> barrel_switcher/12(In10)
  bus_expand1/14(out51) -> barrel_switcher/16(In14)
  bus_expand1/2(out63) -> barrel_switcher/4(In2)
  bus_expand1/60(out5) -> barrel_switcher/62(In60)
  bus_expand1/55(out10) -> barrel_switcher/57(In55)
  bus_expand1/6(out59) -> barrel_switcher/8(In6)
  bus_expand1/47(out18) -> barrel_switcher/49(In47)
  bus_expand1/57(out8) -> barrel_switcher/59(In57)
  bus_expand1/34(out31) -> barrel_switcher/36(In34)
  barrel_switcher/1(sync_out) -> sync_out/1
  bus_create/1(bus_out) -> dout16/1
  barrel_switcher/58(Out57) -> bus_create/1(in1)
  barrel_switcher/59(Out58) -> bus_create/2(in2)
  barrel_switcher/60(Out59) -> bus_create/3(in3)
  barrel_switcher/61(Out60) -> bus_create/4(in4)
  barrel_switcher/62(Out61) -> bus_create/5(in5)
  barrel_switcher/63(Out62) -> bus_create/6(in6)
  barrel_switcher/64(Out63) -> bus_create/7(in7)
  barrel_switcher/65(Out64) -> bus_create/8(in8)

== system c960x4096_x14_7_r2013b_frb/vacc/vacc/xx/bus_expand ==
  bus_in : Inport
  reinterpret{1..16} (16 alike) : xbsIndex_r4/Reinterpret  force_arith_type=on  arith_type="Signed  (2's comp)"  force_bin_pt=on  bin_pt=0  block_type=reinterpret
  slice1 : xbsIndex_r4/Slice  nbits=37  boolean_output=off  mode=Upper Bit Location + Width  bit1=-555  base1=MSB of Input  bit0=0  base0=LSB of Input  dbl_ovrd=off  block_type=slice
  slice10 : xbsIndex_r4/Slice  nbits=37  boolean_output=off  mode=Upper Bit Location + Width  bit1=-222  base1=MSB of Input  bit0=0  base0=LSB of Input  dbl_ovrd=off  block_type=slice
  slice11 : xbsIndex_r4/Slice  nbits=37  boolean_output=off  mode=Upper Bit Location + Width  bit1=-185  base1=MSB of Input  bit0=0  base0=LSB of Input  dbl_ovrd=off  block_type=slice
  slice12 : xbsIndex_r4/Slice  nbits=37  boolean_output=off  mode=Upper Bit Location + Width  bit1=-148  base1=MSB of Input  bit0=0  base0=LSB of Input  dbl_ovrd=off  block_type=slice
  slice13 : xbsIndex_r4/Slice  nbits=37  boolean_output=off  mode=Upper Bit Location + Width  bit1=-111  base1=MSB of Input  bit0=0  base0=LSB of Input  dbl_ovrd=off  block_type=slice
  slice14 : xbsIndex_r4/Slice  nbits=37  boolean_output=off  mode=Upper Bit Location + Width  bit1=-74  base1=MSB of Input  bit0=0  base0=LSB of Input  dbl_ovrd=off  block_type=slice
  slice15 : xbsIndex_r4/Slice  nbits=37  boolean_output=off  mode=Upper Bit Location + Width  bit1=-37  base1=MSB of Input  bit0=0  base0=LSB of Input  dbl_ovrd=off  block_type=slice
  slice16 : xbsIndex_r4/Slice  nbits=37  boolean_output=off  mode=Upper Bit Location + Width  bit1=0  base1=MSB of Input  bit0=0  base0=LSB of Input  dbl_ovrd=off  block_type=slice
  slice2 : xbsIndex_r4/Slice  nbits=37  boolean_output=off  mode=Upper Bit Location + Width  bit1=-518  base1=MSB of Input  bit0=0  base0=LSB of Input  dbl_ovrd=off  block_type=slice
  slice3 : xbsIndex_r4/Slice  nbits=37  boolean_output=off  mode=Upper Bit Location + Width  bit1=-481  base1=MSB of Input  bit0=0  base0=LSB of Input  dbl_ovrd=off  block_type=slice
  slice4 : xbsIndex_r4/Slice  nbits=37  boolean_output=off  mode=Upper Bit Location + Width  bit1=-444  base1=MSB of Input  bit0=0  base0=LSB of Input  dbl_ovrd=off  block_type=slice
  slice5 : xbsIndex_r4/Slice  nbits=37  boolean_output=off  mode=Upper Bit Location + Width  bit1=-407  base1=MSB of Input  bit0=0  base0=LSB of Input  dbl_ovrd=off  block_type=slice
  slice6 : xbsIndex_r4/Slice  nbits=37  boolean_output=off  mode=Upper Bit Location + Width  bit1=-370  base1=MSB of Input  bit0=0  base0=LSB of Input  dbl_ovrd=off  block_type=slice
  slice7 : xbsIndex_r4/Slice  nbits=37  boolean_output=off  mode=Upper Bit Location + Width  bit1=-333  base1=MSB of Input  bit0=0  base0=LSB of Input  dbl_ovrd=off  block_type=slice
  slice8 : xbsIndex_r4/Slice  nbits=37  boolean_output=off  mode=Upper Bit Location + Width  bit1=-296  base1=MSB of Input  bit0=0  base0=LSB of Input  dbl_ovrd=off  block_type=slice
  slice9 : xbsIndex_r4/Slice  nbits=37  boolean_output=off  mode=Upper Bit Location + Width  bit1=-259  base1=MSB of Input  bit0=0  base0=LSB of Input  dbl_ovrd=off  block_type=slice
  msb_out16 : Outport
  out15 : Outport  Port=2
  out14 : Outport  Port=3
  out13 : Outport  Port=4
  out12 : Outport  Port=5
  out11 : Outport  Port=6
  out10 : Outport  Port=7
  out9 : Outport  Port=8
  out8 : Outport  Port=9
  out7 : Outport  Port=10
  out6 : Outport  Port=11
  out5 : Outport  Port=12
  out4 : Outport  Port=13
  out3 : Outport  Port=14
  out2 : Outport  Port=15
  lsb_out1 : Outport  Port=16
  wires:
  bus_in/1 -> slice16/1, slice15/1, slice14/1, slice13/1, slice12/1, slice11/1, slice10/1, slice9/1, slice8/1, slice7/1, slice6/1, slice5/1, slice4/1, slice3/1, slice2/1, slice1/1
  slice16/1 -> reinterpret16/1
  reinterpret16/1 -> msb_out16/1
  slice15/1 -> reinterpret15/1
  reinterpret15/1 -> out15/1
  slice14/1 -> reinterpret14/1
  reinterpret14/1 -> out14/1
  slice13/1 -> reinterpret13/1
  reinterpret13/1 -> out13/1
  slice12/1 -> reinterpret12/1
  reinterpret12/1 -> out12/1
  slice11/1 -> reinterpret11/1
  reinterpret11/1 -> out11/1
  slice10/1 -> reinterpret10/1
  reinterpret10/1 -> out10/1
  slice9/1 -> reinterpret9/1
  reinterpret9/1 -> out9/1
  slice8/1 -> reinterpret8/1
  reinterpret8/1 -> out8/1
  slice7/1 -> reinterpret7/1
  reinterpret7/1 -> out7/1
  slice6/1 -> reinterpret6/1
  reinterpret6/1 -> out6/1
  slice5/1 -> reinterpret5/1
  reinterpret5/1 -> out5/1
  slice4/1 -> reinterpret4/1
  reinterpret4/1 -> out4/1
  slice3/1 -> reinterpret3/1
  reinterpret3/1 -> out3/1
  slice2/1 -> reinterpret2/1
  reinterpret2/1 -> out2/1
  slice1/1 -> reinterpret1/1
  reinterpret1/1 -> lsb_out1/1

== system c960x4096_x14_7_r2013b_frb/vacc/vacc/yy/addr_bram_vacc1 ==
  new_acc : Inport
  din : Inport  Port=2
  Adder : xbsIndex_r4/AddSub  mode=Addition  use_carryin=off  use_carryout=off  en=off  latency=2  precision=User Defined  arith_type="Signed  (2's comp)"  n_bits=n_bits  bin_pt=bin_pt  quantization=Truncate  overflow=Wrap  dbl_ovrd=off  use_behavioral_HDL=on  hw_selection=Fabric  pipelined=off  use_rpm=on  block_type=addsub
      settings: xl_area=[0, 0, 0, 0, 0, 0, 0]  block_version=10.1.3
  Constant : xbsIndex_r4/Constant  const=0  gui_display_data_type=Fixed-point  arith_type=Signed (2's comp)  n_bits=n_bits  bin_pt=bin_pt  preci_type=Single  exp_width=8  frac_width=24  explicit_period=on  period=1  equ=P=C  opselect=C  inp2=PCIN>>17  opr=+  inp1=P  carry=CIN  dbl_ovrd=off  block_type=constant
  Counter : xbsIndex_r4/Counter  cnt_type=Free Running  cnt_to=Inf  operation=Up  start_count=0  cnt_by_val=1  arith_type=Unsigned  n_bits=nextpow2(vec_len)  bin_pt=0  load_pin=off  rst=on  en=off  explicit_period=on  period=1  dbl_ovrd=off  use_behavioral_HDL=on  implementation=Fabric  use_rpm=off  block_type=counter
  Delay1 : xbsIndex_r4/Delay  rst=off  infoeditControl=Selection of Reset will increase slice count due to use of real FFs and instead of SRLs  en=off  latency=1  dbl_ovrd=off  reg_retiming=on  block_type=delay
  Delay2 : xbsIndex_r4/Delay  rst=off  infoeditControl=Selection of Reset will increase slice count due to use of real FFs and instead of SRLs  en=off  latency=1  dbl_ovrd=off  reg_retiming=on  block_type=delay
  Delay4 : xbsIndex_r4/Delay  rst=off  infoeditControl=Selection of Reset will increase slice count due to use of real FFs and instead of SRLs  en=off  latency=1  dbl_ovrd=off  reg_retiming=on  block_type=delay
  Delay8 : xbsIndex_r4/Delay  rst=off  infoeditControl=Selection of Reset will increase slice count due to use of real FFs and instead of SRLs  en=off  latency=2  dbl_ovrd=off  reg_retiming=on  block_type=delay
  Mux : xbsIndex_r4/Mux  inputs=2  en=off  latency=2  precision=Full  arith_type="Signed  (2's comp)"  n_bits=8  bin_pt=2  quantization=Truncate  overflow=Wrap  dbl_ovrd=off  block_type=mux
      settings: xl_area=[0, 0, 0, 0, 0, 0, 0]
  delay_bram : Subsystem  mask(delay_bram){DelayLen=vec_len - 2 - 2, bram_latency=2}
      mask prompts: DelayLen "Delay By:"; bram_latency "BRAM Latency"
      mask help: A delay block that uses BRAM for its storage.
      mask init:
      | if (DelayLen <= bram_latency)
      | 	error('delay value must be greater than BRAM Latency');
      | end
      | BitWidth = max(ceil(log2(DelayLen)), 2);
      mask Help: eval('xlWeb(''http://casper.berkeley.edu/wiki/Delay_bram'')')
  pulse_ext : Subsystem  mask(pulse_ext){pulse_len=vec_len}
      mask prompts: pulse_len "Length of Pulse"
      mask help:
      | Extends a boolean signal to be high for the specified number of clocks after
      | the last high input.
      mask init:
      | bits = ceil(log2(pulse_len+1));
      mask Help: eval('xlWeb(''http://casper.berkeley.edu/wiki/Pulse_ext'')')
  addr : Outport
  dout : Outport  Port=2
  we : Outport  Port=3
  wires:
  Adder/1 -> delay_bram/1(In1)
  delay_bram/1(Out1) -> Mux/2, Delay2/1
  new_acc/1 -> pulse_ext/1(in), Delay4/1
  din/1 -> Delay8/1
  pulse_ext/1(out) -> Mux/1, Delay1/1
  Mux/1 -> Adder/2
  Constant/1 -> Mux/3
  Delay8/1 -> Adder/1
  Counter/1 -> addr/1
  Delay1/1 -> we/1
  Delay2/1 -> dout/1
  Delay4/1 -> Counter/1

== system c960x4096_x14_7_r2013b_frb/vacc/vacc/yy/addr_bram_vacc2 ==
  new_acc : Inport
  din : Inport  Port=2
  Adder : xbsIndex_r4/AddSub  mode=Addition  use_carryin=off  use_carryout=off  en=off  latency=2  precision=User Defined  arith_type="Signed  (2's comp)"  n_bits=n_bits  bin_pt=bin_pt  quantization=Truncate  overflow=Wrap  dbl_ovrd=off  use_behavioral_HDL=on  hw_selection=Fabric  pipelined=off  use_rpm=on  block_type=addsub
      settings: xl_area=[0, 0, 0, 0, 0, 0, 0]  block_version=10.1.3
  Constant : xbsIndex_r4/Constant  const=0  gui_display_data_type=Fixed-point  arith_type=Signed (2's comp)  n_bits=n_bits  bin_pt=bin_pt  preci_type=Single  exp_width=8  frac_width=24  explicit_period=on  period=1  equ=P=C  opselect=C  inp2=PCIN>>17  opr=+  inp1=P  carry=CIN  dbl_ovrd=off  block_type=constant
  Counter : xbsIndex_r4/Counter  cnt_type=Free Running  cnt_to=Inf  operation=Up  start_count=0  cnt_by_val=1  arith_type=Unsigned  n_bits=nextpow2(vec_len)  bin_pt=0  load_pin=off  rst=on  en=off  explicit_period=on  period=1  dbl_ovrd=off  use_behavioral_HDL=on  implementation=Fabric  use_rpm=off  block_type=counter
  Delay1 : xbsIndex_r4/Delay  rst=off  infoeditControl=Selection of Reset will increase slice count due to use of real FFs and instead of SRLs  en=off  latency=1  dbl_ovrd=off  reg_retiming=on  block_type=delay
  Delay2 : xbsIndex_r4/Delay  rst=off  infoeditControl=Selection of Reset will increase slice count due to use of real FFs and instead of SRLs  en=off  latency=1  dbl_ovrd=off  reg_retiming=on  block_type=delay
  Delay4 : xbsIndex_r4/Delay  rst=off  infoeditControl=Selection of Reset will increase slice count due to use of real FFs and instead of SRLs  en=off  latency=1  dbl_ovrd=off  reg_retiming=on  block_type=delay
  Delay8 : xbsIndex_r4/Delay  rst=off  infoeditControl=Selection of Reset will increase slice count due to use of real FFs and instead of SRLs  en=off  latency=2  dbl_ovrd=off  reg_retiming=on  block_type=delay
  Mux : xbsIndex_r4/Mux  inputs=2  en=off  latency=2  precision=Full  arith_type="Signed  (2's comp)"  n_bits=8  bin_pt=2  quantization=Truncate  overflow=Wrap  dbl_ovrd=off  block_type=mux
      settings: xl_area=[0, 0, 0, 0, 0, 0, 0]
  delay_bram : Subsystem  mask(delay_bram){DelayLen=vec_len - 2 - 2, bram_latency=2}
      mask prompts: DelayLen "Delay By:"; bram_latency "BRAM Latency"
      mask help: A delay block that uses BRAM for its storage.
      mask init:
      | if (DelayLen <= bram_latency)
      | 	error('delay value must be greater than BRAM Latency');
      | end
      | BitWidth = max(ceil(log2(DelayLen)), 2);
      mask Help: eval('xlWeb(''http://casper.berkeley.edu/wiki/Delay_bram'')')
  pulse_ext : Subsystem  mask(pulse_ext){pulse_len=vec_len}
      mask prompts: pulse_len "Length of Pulse"
      mask help:
      | Extends a boolean signal to be high for the specified number of clocks after
      | the last high input.
      mask init:
      | bits = ceil(log2(pulse_len+1));
      mask Help: eval('xlWeb(''http://casper.berkeley.edu/wiki/Pulse_ext'')')
  addr : Outport
  dout : Outport  Port=2
  we : Outport  Port=3
  wires:
  Adder/1 -> delay_bram/1(In1)
  delay_bram/1(Out1) -> Mux/2, Delay2/1
  new_acc/1 -> pulse_ext/1(in), Delay4/1
  din/1 -> Delay8/1
  pulse_ext/1(out) -> Mux/1, Delay1/1
  Mux/1 -> Adder/2
  Constant/1 -> Mux/3
  Delay8/1 -> Adder/1
  Counter/1 -> addr/1
  Delay1/1 -> we/1
  Delay2/1 -> dout/1
  Delay4/1 -> Counter/1
